simulink model "SendString"  (R2018a)
settings: Solver=VariableStepAuto  StartTime=0.0  StopTime=inf  RelTol=1e-3
libraries: powerlib_meascontrol x2, svdutilitieslib x2, xpcrtudplib x2, aerolibanimutils x1
settings Model: NumberOfSteps=10  Creator=gyga  LastModifiedBy=gyga

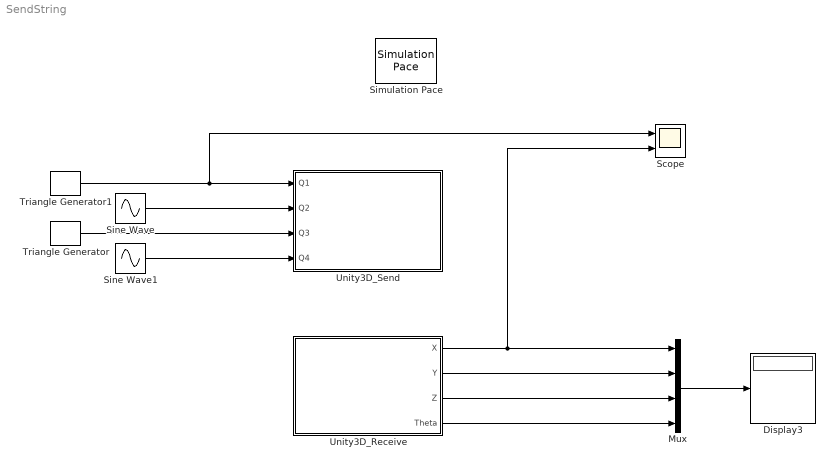
== system SendString ==
  Display3 : Display
  Mux : Mux
  Scope : Scope  NumInputPorts=2
  Simulation Pace : aerolibanimutils/Simulation Pace  SimulationPace=1  SleepMode=MATLAB Thread  OutputPaceError=off  SampleTime=1/100
  Sine Wave : Sin  Frequency=1*2*pi  SampleTime=0
  Sine Wave1 : Sin  Frequency=.75*2*pi  SampleTime=0
  Triangle Generator : powerlib_meascontrol/Pulse & Signal Generators/Triangle Generator  Freq=1  Phase=90  Ts=0
  Triangle Generator1 : powerlib_meascontrol/Pulse & Signal Generators/Triangle Generator  Freq=.5  Phase=90  Ts=0
  Unity3D_Receive : Subsystem
      mask Display: disp('Receive from Unity3D')
  Unity3D_Send : Subsystem
      mask Display: disp('Send To Unity3D');
  wires:
  Triangle Generator1/1 -> Scope/1, Unity3D_Send/1(Q1)
  Mux/1 -> Display3/1
  Sine Wave/1 -> Unity3D_Send/2(Q2)
  Triangle Generator/1 -> Unity3D_Send/3(Q3)
  Sine Wave1/1 -> Unity3D_Send/4(Q4)
  Unity3D_Receive/1(X) -> Mux/1, Scope/2
  Unity3D_Receive/2(Y) -> Mux/2
  Unity3D_Receive/3(Z) -> Mux/3
  Unity3D_Receive/4(Theta) -> Mux/4

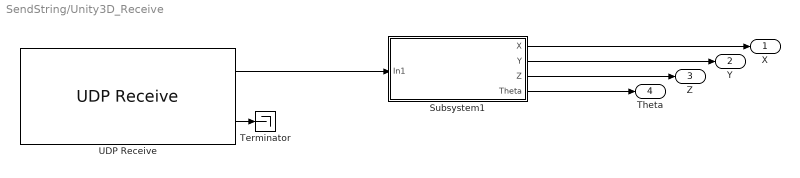
== system SendString/Unity3D_Receive ==
  Subsystem1 : Subsystem
      mask Display: disp('String To Data')
  Terminator : Terminator
  UDP Receive : xpcrtudplib/UDP Receive  ipAddressVal=Use host-target connection  localPort=25005  rcvWidth=60  rcvFmAny=on  fmAddress=0.0.0.0  rcvMulticast=off  multicastAddress=[]  maxUDPQueue=8  sampleTime=-1
      settings: SourceProductName=Simulink Real-Time
  X : Outport
  Y : Outport  Port=2
  Z : Outport  Port=3
  Theta : Outport  Port=4
  wires:
  UDP Receive/2 -> Terminator/1
  Subsystem1/2(Y) -> Y/1
  Subsystem1/1(X) -> X/1
  Subsystem1/3(Z) -> Z/1
  Subsystem1/4(Theta) -> Theta/1
  UDP Receive/1 -> Subsystem1/1(In1)

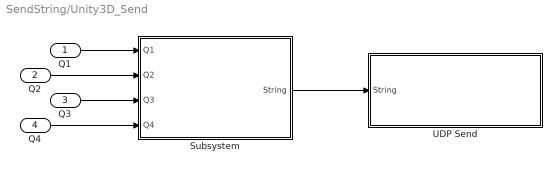
== system SendString/Unity3D_Send ==
  Q1 : Inport
  Q2 : Inport  Port=2
  Q3 : Inport  Port=3
  Q4 : Inport  Port=4
  Subsystem : Subsystem
      mask Display: disp('Data to String');
  UDP Send : Subsystem  mask{IP='127.0.0.1', LocalPort=25001, ToPort=25002, MaxLength=60}
      mask prompts: IP "IP addres"; LocalPort "From port"; ToPort "To port"; MaxLength "Max length"
      mask Display:
      | ToPort = get_param(gcb, 'ToPort');
      | LocalPort = get_param(gcb, 'LocalPort');
      | IP = get_param(gcb, 'IP');
      | % str = sprintf('UDP String Send\nFrom port: \nTo port: \n');
      | % fprintf(str);
      | text(49, 57, 'UDP String Send')
      | text(49, 57-15, 'IP:')
      | text(49, 57-2*15, 'From Port:')
      | text(49, 57-3*15, 'To Port:')
      | 
      | color('blue');
      | 
      | text(64, 57-15, IP)
      | text(100, 57-2*15, LocalPort)
      | text(87, 57-3*15, ToPort)
  wires:
  Q4/1 -> Subsystem/4(Q4)
  Q3/1 -> Subsystem/3(Q3)
  Subsystem/1(String) -> UDP Send/1(String)
  Q1/1 -> Subsystem/1(Q1)
  Q2/1 -> Subsystem/2(Q2)

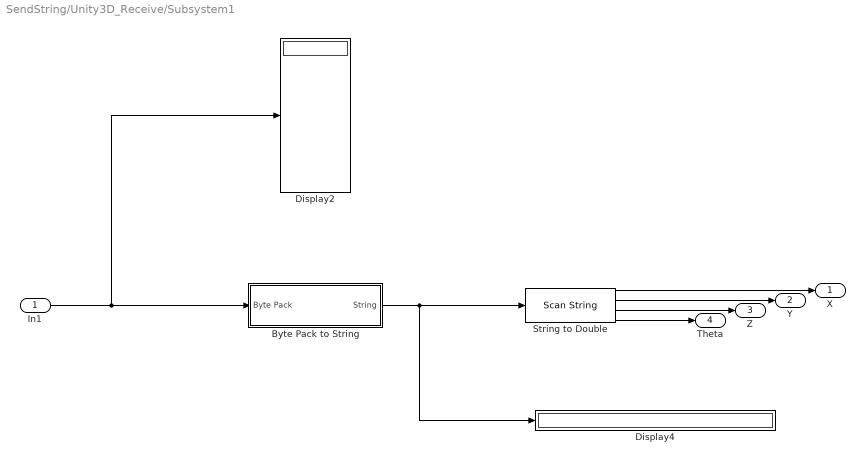
== system SendString/Unity3D_Receive/Subsystem1 ==
  In1 : Inport
  Byte Pack to String : Subsystem
  Display2 : Display
  Display4 : Display
  String to Double : ScanString  Format="\"%f %f %f %f\""
  X : Outport
  Y : Outport  Port=2
  Z : Outport  Port=3
  Theta : Outport  Port=4
  wires:
  String to Double/4 -> Theta/1
  String to Double/2 -> Y/1
  Byte Pack to String/1(String) -> String to Double/1, Display4/1
  String to Double/3 -> Z/1
  In1/1 -> Byte Pack to String/1(Byte Pack), Display2/1
  String to Double/1 -> X/1

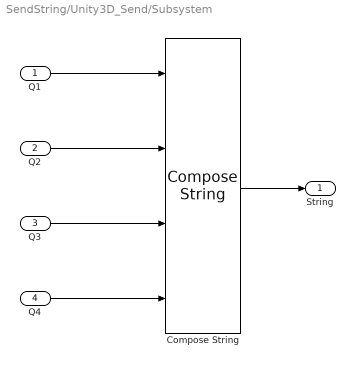
== system SendString/Unity3D_Send/Subsystem ==
  Q1 : Inport
  Q2 : Inport  Port=2
  Q3 : Inport  Port=3
  Q4 : Inport  Port=4
  Compose String : ComposeString  Format="\"%.2f %.2f %.2f %.2f\""
  String : Outport
  wires:
  Q1/1 -> Compose String/1
  Q3/1 -> Compose String/3
  Q2/1 -> Compose String/2
  Compose String/1 -> String/1
  Q4/1 -> Compose String/4

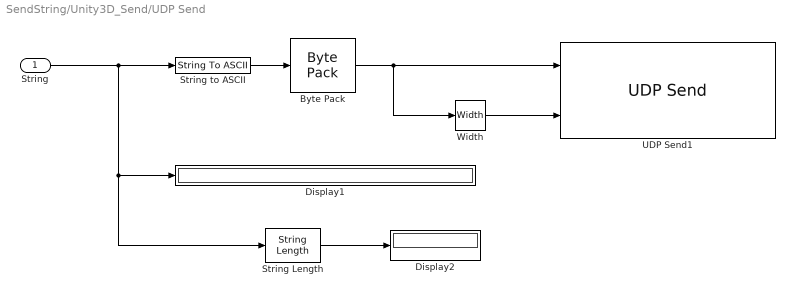
== system SendString/Unity3D_Send/UDP Send ==
  String : Inport
  Byte Pack : svdutilitieslib/Byte Pack  maskPackedDataType=uint8  datatypes={'uint8'}  byteAlign=1  blockPlatform=arduinoert
      settings: SourceProductName=Simulink Support Package for Arduino Hardware  SourceProductBaseCode=ARDUINO
  Display1 : Display
  Display2 : Display
  String Length : StringLength
  String to ASCII : StringToASCII  MaximumLength=60
  UDP Send1 : xpcrtudplib/UDP Send  ipAddressVal=Use host-target connection  localPort=LocalPort  toAddress=IP  toPort=ToPort  sampleTime=-1
      settings: SourceProductName=Simulink Real-Time  SourceProductBaseCode=XP
  Width : Width
  wires:
  Width/1 -> UDP Send1/2
  Byte Pack/1 -> UDP Send1/1, Width/1
  String to ASCII/1 -> Byte Pack/1
  String Length/1 -> Display2/1
  String/1 -> String Length/1, Display1/1, String to ASCII/1

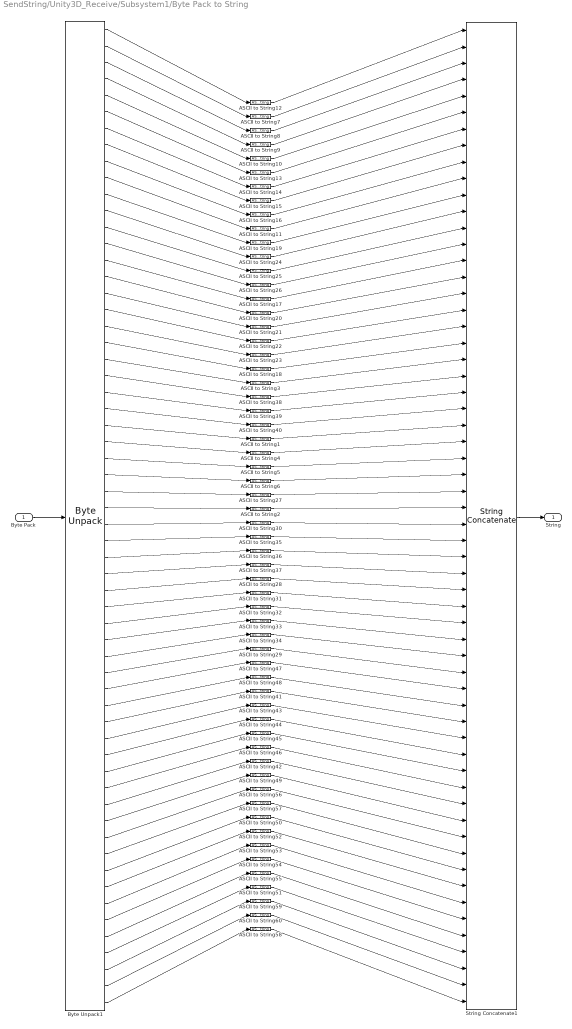
== system SendString/Unity3D_Receive/Subsystem1/Byte Pack to String ==
  Byte Pack : Inport
  ASCII to String{1..60} (60 alike) : ASCIIToString
  Byte Unpack1 : svdutilitieslib/Byte Unpack  dimensions={1, 1, 1, 1, 1, 1, 1, 1, 1, 1, 1, 1, 1, 1, 1, 1, 1, 1, 1, 1, 1, 1, 1, 1, 1, 1, 1, 1, 1, 1, 1, 1, 1, 1, 1, 1, 1, 1, 1, 1, 1, 1, 1, 1, 1, 1, 1, 1, 1, 1, 1, 1, 1, 1, 1, 1, 1, 1, 1, 1}  datatypes={'uint8', 'uint8', 'uint8', 'uint8', 'uint8', 'uint8', 'uint8', 'uint8', 'uint8', 'uint8', 'uint8', 'uint8', 'uint8', 'uint8', 'uint8', 'uint8', 'uint8', 'uint8', 'uint8', 'uint8', 'uint8', 'uint8', 'uint8', 'uint8', 'uint8', 'uint8', 'uint8', 'uint8', 'uint8', 'uint8', 'uint8', 'uint8', 'uint8', 'uint8', 'uint8', 'uint8', 'uint8', 'uint8', 'uint8', 'uint8', 'uint8', 'uint8', 'uint8', 'uint8', 'uint8', 'uint8', 'uint8', 'uint8', 'uint8', 'uint8', 'uint8', 'uint8', 'uint8', 'uint8', 'uint8', 'uint8', 'uint8', 'uint8', 'uint8', 'uint8'}  byteAlign=1  blockPlatform=arduinoert
      settings: SourceProductName=Simulink Support Package for Arduino Hardware  SourceProductBaseCode=ARDUINO
  String Concatenate1 : StringConcatenate  Inputs=60
  String : Outport
  wires:
  Byte Unpack1/9 -> ASCII to String16/1
  ASCII to String8/1 -> String Concatenate1/3
  Byte Unpack1/2 -> ASCII to String7/1
  Byte Unpack1/5 -> ASCII to String10/1
  ASCII to String24/1 -> String Concatenate1/12
  ASCII to String16/1 -> String Concatenate1/9
  Byte Unpack1/4 -> ASCII to String9/1
  Byte Unpack1/1 -> ASCII to String12/1
  ASCII to String1/1 -> String Concatenate1/25
  ASCII to String20/1 -> String Concatenate1/16
  Byte Unpack1/11 -> ASCII to String19/1
  Byte Unpack1/17 -> ASCII to String21/1
  ASCII to String22/1 -> String Concatenate1/18
  ASCII to String12/1 -> String Concatenate1/1
  ASCII to String19/1 -> String Concatenate1/11
  ASCII to String15/1 -> String Concatenate1/8
  ASCII to String43/1 -> String Concatenate1/44
  ASCII to String14/1 -> String Concatenate1/7
  Byte Unpack1/8 -> ASCII to String15/1
  ASCII to String7/1 -> String Concatenate1/2
  ASCII to String26/1 -> String Concatenate1/14
  Byte Unpack1/15 -> ASCII to String17/1
  Byte Unpack1/7 -> ASCII to String14/1
  Byte Unpack1/13 -> ASCII to String25/1
  ASCII to String33/1 -> String Concatenate1/38
  Byte Unpack1/10 -> ASCII to String11/1
  ASCII to String23/1 -> String Concatenate1/19
  ASCII to String11/1 -> String Concatenate1/10
  ASCII to String37/1 -> String Concatenate1/34
  Byte Unpack1/20 -> ASCII to String18/1
  Byte Unpack1/19 -> ASCII to String23/1
  Byte Unpack1/16 -> ASCII to String20/1
  ASCII to String40/1 -> String Concatenate1/24
  ASCII to String13/1 -> String Concatenate1/6
  Byte Unpack1/14 -> ASCII to String26/1
  ASCII to String18/1 -> String Concatenate1/20
  Byte Unpack1/6 -> ASCII to String13/1
  Byte Unpack1/12 -> ASCII to String24/1
  Byte Unpack1/3 -> ASCII to String8/1
  ASCII to String47/1 -> String Concatenate1/41
  Byte Unpack1/18 -> ASCII to String22/1
  ASCII to String25/1 -> String Concatenate1/13
  ASCII to String3/1 -> String Concatenate1/21
  ASCII to String39/1 -> String Concatenate1/23
  ASCII to String17/1 -> String Concatenate1/15
  ASCII to String21/1 -> String Concatenate1/17
  ASCII to String5/1 -> String Concatenate1/27
  ASCII to String9/1 -> String Concatenate1/4
  ASCII to String28/1 -> String Concatenate1/35
  ASCII to String10/1 -> String Concatenate1/5
  ASCII to String42/1 -> String Concatenate1/48
  ASCII to String41/1 -> String Concatenate1/43
  ASCII to String34/1 -> String Concatenate1/39
  ASCII to String4/1 -> String Concatenate1/26
  ASCII to String32/1 -> String Concatenate1/37
  ASCII to String29/1 -> String Concatenate1/40
  ASCII to String48/1 -> String Concatenate1/42
  ASCII to String27/1 -> String Concatenate1/29
  ASCII to String44/1 -> String Concatenate1/45
  Byte Pack/1 -> Byte Unpack1/1
  ASCII to String35/1 -> String Concatenate1/32
  ASCII to String2/1 -> String Concatenate1/30
  ASCII to String38/1 -> String Concatenate1/22
  ASCII to String36/1 -> String Concatenate1/33
  ASCII to String46/1 -> String Concatenate1/47
  ASCII to String31/1 -> String Concatenate1/36
  ASCII to String45/1 -> String Concatenate1/46
  ASCII to String30/1 -> String Concatenate1/31
  ASCII to String6/1 -> String Concatenate1/28
  Byte Unpack1/38 -> ASCII to String33/1
  Byte Unpack1/23 -> ASCII to String39/1
  Byte Unpack1/32 -> ASCII to String35/1
  Byte Unpack1/26 -> ASCII to String4/1
  Byte Unpack1/34 -> ASCII to String37/1
  Byte Unpack1/36 -> ASCII to String31/1
  Byte Unpack1/39 -> ASCII to String34/1
  Byte Unpack1/40 -> ASCII to String29/1
  Byte Unpack1/30 -> ASCII to String2/1
  Byte Unpack1/33 -> ASCII to String36/1
  Byte Unpack1/27 -> ASCII to String5/1
  Byte Unpack1/35 -> ASCII to String28/1
  Byte Unpack1/28 -> ASCII to String6/1
  Byte Unpack1/37 -> ASCII to String32/1
  Byte Unpack1/31 -> ASCII to String30/1
  Byte Unpack1/21 -> ASCII to String3/1
  Byte Unpack1/24 -> ASCII to String40/1
  Byte Unpack1/25 -> ASCII to String1/1
  Byte Unpack1/22 -> ASCII to String38/1
  Byte Unpack1/29 -> ASCII to String27/1
  String Concatenate1/1 -> String/1
  Byte Unpack1/45 -> ASCII to String44/1
  Byte Unpack1/43 -> ASCII to String41/1
  Byte Unpack1/41 -> ASCII to String47/1
  Byte Unpack1/48 -> ASCII to String42/1
  Byte Unpack1/47 -> ASCII to String46/1
  Byte Unpack1/44 -> ASCII to String43/1
  Byte Unpack1/42 -> ASCII to String48/1
  Byte Unpack1/46 -> ASCII to String45/1
  Byte Unpack1/55 -> ASCII to String54/1
  Byte Unpack1/51 -> ASCII to String57/1
  Byte Unpack1/53 -> ASCII to String52/1
  Byte Unpack1/56 -> ASCII to String55/1
  Byte Unpack1/57 -> ASCII to String51/1
  Byte Unpack1/50 -> ASCII to String56/1
  Byte Unpack1/52 -> ASCII to String50/1
  Byte Unpack1/54 -> ASCII to String53/1
  Byte Unpack1/49 -> ASCII to String49/1
  ASCII to String54/1 -> String Concatenate1/55
  ASCII to String55/1 -> String Concatenate1/56
  ASCII to String53/1 -> String Concatenate1/54
  ASCII to String57/1 -> String Concatenate1/51
  ASCII to String49/1 -> String Concatenate1/49
  ASCII to String50/1 -> String Concatenate1/52
  ASCII to String51/1 -> String Concatenate1/57
  ASCII to String56/1 -> String Concatenate1/50
  ASCII to String52/1 -> String Concatenate1/53
  ASCII to String58/1 -> String Concatenate1/60
  ASCII to String60/1 -> String Concatenate1/59
  ASCII to String59/1 -> String Concatenate1/58
  Byte Unpack1/60 -> ASCII to String58/1
  Byte Unpack1/59 -> ASCII to String60/1
  Byte Unpack1/58 -> ASCII to String59/1
